simulink model "hpa_module"  (R2020a)
settings: Solver=FixedStepDiscrete  StartTime=0.0  StopTime=inf  RelTol=1e-3
InitFcn:
  | f = 300e6;
libraries: hdlsllib x3, simulink x1
settings Model: DataTypeOverride=Off  Creator=David Northcote  LastModifiedBy=david
settings DataIOCC: SaveOutput=off  SaveTime=off
settings OptimizationCC: BlockReduction=off  ConditionallyExecuteInputs=off  DefaultParameterBehavior=Inlined
settings DebuggingCC: AlgebraicLoopMsg=error  SingleTaskRateTransMsg=error
settings HardwareCC: ProdBitPerPointer=32  ProdBitPerSizeT=32  ProdBitPerPtrDiffT=32  ProdLargestAtomicFloat=None  ProdIntDivRoundTo=Undefined  ProdEndianess=Unspecified  ProdWordSize=32  ProdHWDeviceType=ASIC/FPGA->ASIC/FPGA  TargetBitPerPointer=64  TargetBitPerSizeT=64  TargetBitPerPtrDiffT=64  TargetLongLongMode=on  TargetIntDivRoundTo=Zero  TargetEndianess=LittleEndian  TargetWordSize=64  TargetHWDeviceType=Custom Processor->MATLAB Host Computer  ProdEqTarget=off
settings SFSimCC: CustomCodeUndefinedFunction=UseInterfaceOnly

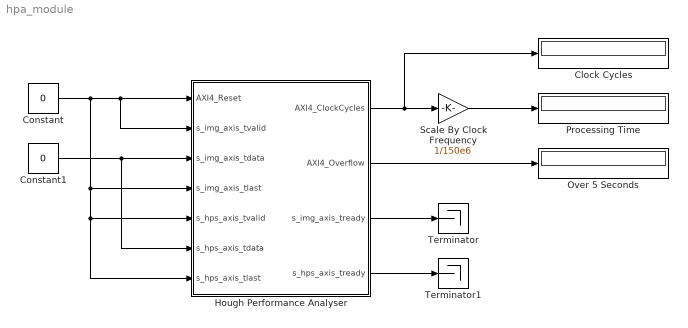
== system hpa_module ==
  Clock Cycles : Display
  Constant : Constant  Value=0  OutDataTypeStr=boolean  SampleTime=1/150e6
  Constant1 : Constant  Value=0  OutDataTypeStr=uint32  SampleTime=1/150e6
  Hough Performance Analyser : Subsystem  TreatAsAtomicUnit=on
  Over 5 Seconds : Display
  Processing Time : Display
  Scale By Clock Frequency : Gain  Gain=1/150e6
  Terminator : Terminator
  Terminator1 : Terminator
  wires:
  Constant/1 -> Hough Performance Analyser/1(AXI4_Reset), Hough Performance Analyser/2(s_img_axis_tvalid), Hough Performance Analyser/7(s_hps_axis_tlast), Hough Performance Analyser/5(s_hps_axis_tvalid), Hough Performance Analyser/4(s_img_axis_tlast)
  Hough Performance Analyser/2(AXI4_Overflow) -> Over 5 Seconds/1
  Scale By Clock Frequency/1 -> Processing Time/1
  Hough Performance Analyser/1(AXI4_ClockCycles) -> Clock Cycles/1, Scale By Clock Frequency/1
  Constant1/1 -> Hough Performance Analyser/6(s_hps_axis_tdata), Hough Performance Analyser/3(s_img_axis_tdata)
  Hough Performance Analyser/3(s_img_axis_tready) -> Terminator/1
  Hough Performance Analyser/4(s_hps_axis_tready) -> Terminator1/1

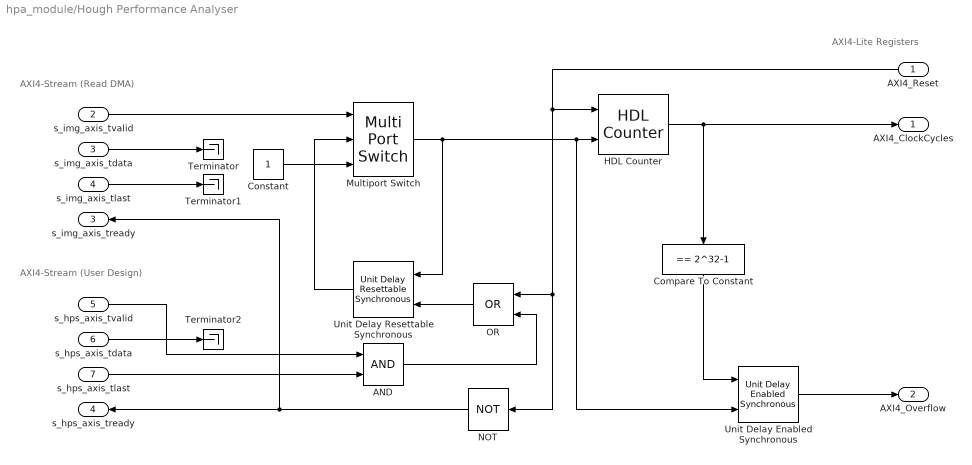
== system hpa_module/Hough Performance Analyser ==
  note: AXI4-Lite Registers
  note: AXI4-Stream (User Design)
  note: AXI4-Stream (Read DMA)
  AXI4_Reset : Inport
  s_img_axis_tvalid : Inport  Port=2
  s_img_axis_tdata : Inport  Port=3
  s_img_axis_tlast : Inport  Port=4
  s_hps_axis_tvalid : Inport  Port=5
  s_hps_axis_tdata : Inport  Port=6
  s_hps_axis_tlast : Inport  Port=7
  AND : Logic  IconShape=distinctive  AllPortsSameDT=off  OutDataTypeStr=boolean
  Compare To Constant : simulink/Logic and Bit Operations/Compare To Constant  relop===  const=2^32-1  OutDataTypeStr=boolean
  Constant : Constant  OutDataTypeStr=boolean  SampleTime=-1
  HDL Counter : hdlsllib/Sources/HDL Counter  CountType=Count limited  CountInit=0  CountStep=1  CountMax=2^32-1  CountFromType=Initial value  CountFrom=0  CountResetPort=on  CountLoadPort=off  CountEnbPort=on  CountDirPort=off  CountDataType=Unsigned  CountWordLen=32  CountFracLen=0  CountSampTime=1
  Multiport Switch : MultiPortSwitch  DataPortOrder=Zero-based contiguous  Inputs=2  zeroidx=on
  NOT : Logic  Operator=NOT  IconShape=distinctive  AllPortsSameDT=off  OutDataTypeStr=boolean
  OR : Logic  Operator=OR  IconShape=distinctive  AllPortsSameDT=off  OutDataTypeStr=boolean
  Terminator : Terminator
  Terminator1 : Terminator
  Terminator2 : Terminator
  Unit Delay Enabled Synchronous : hdlsllib/Discrete/Unit Delay Enabled Synchronous  InitialCondition=0.0  SampleTime=-1
      settings: SourceProductBaseCode=SL
  Unit Delay Resettable Synchronous : hdlsllib/Discrete/Unit Delay Resettable Synchronous  InitialCondition=0.0  SampleTime=-1
      settings: SourceProductBaseCode=SL
  AXI4_ClockCycles : Outport
  AXI4_Overflow : Outport  Port=2
  s_img_axis_tready : Outport  Port=3
  s_hps_axis_tready : Outport  Port=4
  wires:
  Constant/1 -> Multiport Switch/3
  Unit Delay Resettable Synchronous/1 -> Multiport Switch/2
  Multiport Switch/1 -> Unit Delay Resettable Synchronous/1, Unit Delay Enabled Synchronous/2, HDL Counter/2
  Compare To Constant/1 -> Unit Delay Enabled Synchronous/1
  Unit Delay Enabled Synchronous/1 -> AXI4_Overflow/1
  HDL Counter/1 -> Compare To Constant/1, AXI4_ClockCycles/1
  s_hps_axis_tdata/1 -> Terminator2/1
  s_img_axis_tdata/1 -> Terminator/1
  AXI4_Reset/1 -> NOT/1, OR/1, HDL Counter/1
  s_img_axis_tlast/1 -> Terminator1/1
  OR/1 -> Unit Delay Resettable Synchronous/2
  s_img_axis_tvalid/1 -> Multiport Switch/1
  AND/1 -> OR/2
  s_hps_axis_tlast/1 -> AND/2
  s_hps_axis_tvalid/1 -> AND/1
  NOT/1 -> s_img_axis_tready/1, s_hps_axis_tready/1
